simulink model "sis_electromecanicos_simulink"  (R2023b)
settings: Solver=VariableStepAuto  StartTime=0.0  StopTime=10.0  RelTol=1e-3
settings Model: Creator=penqu  LastModifiedBy=penqu

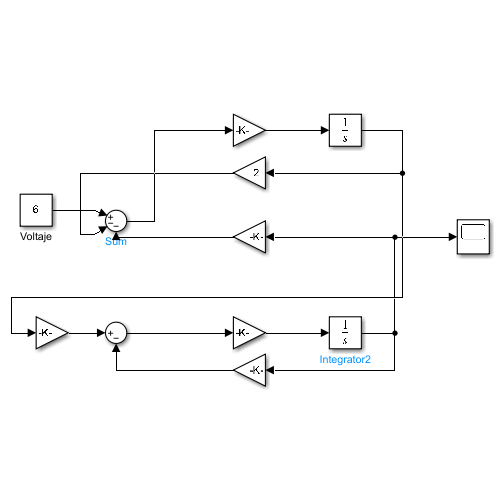
[thumbnail: Simulink's stored preview of the top-level diagram]
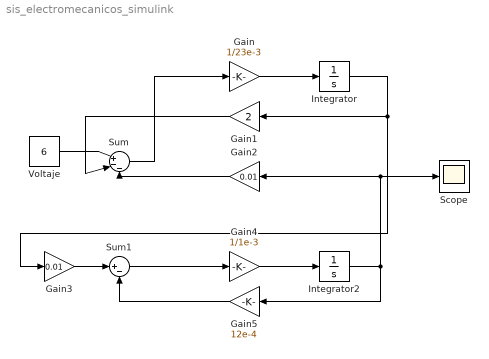
== system sis_electromecanicos_simulink ==
  Gain : Gain  Gain=1/23e-3
  Gain1 : Gain  Gain=2
  Gain2 : Gain  Gain=0.01
  Gain3 : Gain  Gain=0.01
  Gain4 : Gain  Gain=1/1e-3
  Gain5 : Gain  Gain=12e-4
  Integrator : Integrator
  Integrator2 : Integrator
  Scope : Scope
  Sum : Sum  Inputs=|+--
  Sum1 : Sum  Inputs=|+-
  Voltaje : Constant  Value=6
  wires:
  Gain1/1 -> Sum/2
  Gain4/1 -> Integrator2/1
  Gain5/1 -> Sum1/2
  Sum1/1 -> Gain4/1
  Integrator2/1 -> Gain5/1, Scope/1, Gain2/1
  Gain2/1 -> Sum/3
  Gain3/1 -> Sum1/1
  Sum/1 -> Gain/1
  Gain/1 -> Integrator/1
  Integrator/1 -> Gain3/1, Gain1/1
  Voltaje/1 -> Sum/1
